simulink model "CDC_Library"  (R2015b)
settings: Solver=VariableStepAuto  StartTime=0  StopTime=1296000  RelTol=1e-3
InitFcn:
  | CD2_init
undefined symbols (not defined in the file): CD2_get_substances_count, table, tablestep
libraries: simulink x1
settings Model: Creator=garbanlo  LastModifiedBy=garbanlo
settings DataIOCC: LimitDataPoints=off  TimeSaveName=cd_time

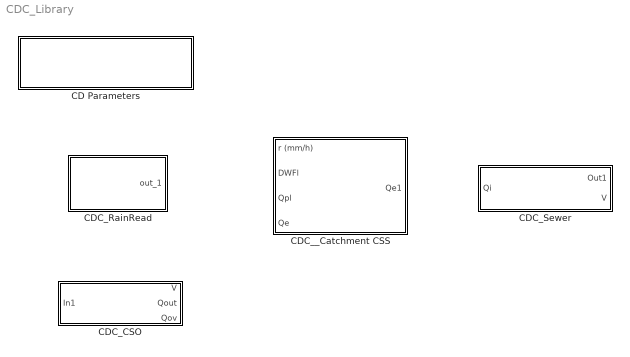
== system CDC_Library ==
  CD Parameters : Subsystem  mask(City Drain 2.0 - Simulation parameters){subst='COD HCO3 NH4', t_step=0, t_start=0, t_stop=15*24*60*60}
      mask prompts: subst "Modell Substances list (string)"; t_step "Sampling Time [s]"; t_start "Start Time [s]"; t_stop "Stop Time [s]"
      mask help:
      | Block that sets the global parameters required in City Drain 2.0. Following paramters are set without user's input:
      |
      | - 'Solver' --> 'FixedStepDiscrete'
      | - 'TimeSaveName' --> 'cd_time'
      | - 'Decimation' --> '1'
      | - 'LimitDataPoints' -->  'off'
      mask init:
      | % toplevel systems' name --> Plant file name;
      | tls=bdroot(gcb); 
      | %set_param(tls, 'Solver', 'FixedStepDiscrete'); 
      | set_param(tls, 'TimeSaveName', 'cd_time');
      | set_param(tls, 'Decimation', '1');
      | set_param(tls, 'LimitDataPoints', 'off');
      | set_param(tls, 'ScreenColor', 'white');
      | 
      | %tstep_char=num2str(t_step); % Setting the discrete time step
      | % set_param(tls, 'FixedStep', tstep_char); 
      | 
      | tstart_char=num2str(t_start); % Setting the start time
      | set_param(tls, 'StartTime', tstart_char); 
      | 
      | tstop_char=num2str(t_stop); % Setting the stop time
      | set_param(tls, 'StopTime', tstop_char);
      | 
      | set_param(gcs,'InitFcn','CD2_init');
      mask Display:
      | plot(0,0,100,100);
      | 
      | text(50,65,'CITY DRAIN','HorizontalAlignment','center');
      | text(50,35,'PARAMETERS','HorizontalAlignment','center');
      | 
      | 
      | image(imread('CityDrain_SimParam.jpg'))
  CDC_CSO : Subsystem  mask{Qout=0.02, V=1000, n_comp=CD2_get_substances_count}
      mask prompts: Qout "maximum outflow"; V "volume [m^3]"; n_comp "number of pollutants"
  CDC_RainRead : Subsystem  mask(Rain Read){table0='rainPulse5min.ixx', crep=off}
      mask prompts: table0 "Filename"; crep "Cylic repitition"
      mask help:
      | Read raindata from ASCII File in following formats:
      |
      | *.ixx ... Format used by the Austrian Hydrographic Service.
      | *.km2 ... Format used in the Mouse Software from DHI (Danish Hydraulic Institute)
      | *.mse ... modified mse format used in  Mouse Software from DHI (Danish Hydraulic Institute)
      |
      | Used function: CD1_mfun_rainread.m
      mask init:
      | % cache table size set to 1000
      | %table=zeros(1000,2)
      | [table,tablestep]=CD1_mfun_rainread(table0);
      | 
      | % reading the toplevel systems' name 
      | % --> Plant file name;
      | tls=bdroot(gcb); 
      | % Obtaining the fixed sampling time
      | % t_samp_char=get_param(tls, 'FixedStep');
      | % Convertion to numeric value
      | tstep = -1;
      mask Display:
      | plot(0,0,100,100);
      | 
      | text(40,40,'RAIN READ');
      | plot( [5 10 10 15 15 20 20 25 25 30 30 40 40 45], [0 0 20 20 40 40 60 60 30 30 0 0 0 0]+20);
  CDC_Sewer : Subsystem  mask(Sewer){K=300, alpha=0.5, n_comp=CD2_get_substances_count, beta=0.0001}
      mask prompts: K "K (travel time) [s]"; alpha "alpha (weighing factor,  0-1)  [ - ]"; n_comp "Number of pollutants [ - ]"; beta "beta (weighting factor)"
      mask help:
      | Function used:
      | CD1_sfun_Muskingum_Sewer.m
      mask init:
      | %arrow location in icon
      | kx=70;
      | ky=25;
      | % picture location
      | x=20;y=25;
      | 
      | 
      | % reading the toplevel systems' name 
      | % --> Plant file name;
      | % tls=bdroot(gcb); 
      | % Obtaining the fixed sampling time
      | % t_samp_char=get_param(tls, 'FixedStep');
      | % Convertion to numeric value
      | % dt = str2num(t_samp_char); 
      | tstep = -11
      mask Display:
      | plot(0,0,100,50, [0,50,50,0,0]+x,[-10,-10,10,10,-10]+y, [10,10]+x,[-10,10]+y, [20,20]+x,[-10,10]+y, [30,30]+x,[-10,10]+y, [40,40]+x,[-10,10]+y, [0,0,5,5,10,5,5,0]+kx, [5,-5,-5,-13,0,13,5,5]+ky );
      | 
      | 
      | text(50,7,'SEWER sM','HorizontalAlignment','center');
      | 
      | port_label('input',1,'Qi');
      | port_label('output',1,'Qe');
      | port_label('output',2,'VCi');
  CDC__Catchment CSS : Subsystem  mask(Catchment CSS){area=2, rfcoeff=0.5, initloss=1.5, permloss=1.25, N=3, n_comp=CD2_get_substances_count, Rain_C=[2 0 0], K=300, X=0}
      mask prompts: area "Area in [ha]"; rfcoeff "Runoff coefficient (0 - 1)"; initloss "Initial Loss in [mm]"; permloss "Permanent loss in [mm/day]"; N "No of Timesteps (transport time) / No of subareas n [-]"; n_comp "No of pollutant components"; Rain_C "Vector of Rain-Conc. [g/m3]"
      mask help:
      | Hydrological model of an urban catchment with a combined sewer system.
      | --> see manual for more details
      mask init:
      | % location of catchment drawing
      | x=10;
      | y=-10;
      | % reading the toplevel systems' name 
      | % --> Plant file name;
      | tls=bdroot(gcb); 
      | % Obtaining the fixed sampling time
      | % t_samp_char=get_param(tls, 'FixedStep');
      | 
      | % Convertion to numeric value
      | % tstep = str2num(t_samp_char); 
      | tstep = 60;
      | 
      | %convertion form mm/day --> mm/s
      | permloss=permloss/86400;
      | area=area*10000;
      | 
      | %parameter for muskingum
      | CX=(-K*X)/(K*(1-X));
      | CY=1/(K*(1-X));
      mask Display:
      | plot(0,0,100,100, [17 20 25 30 40 45 50 55 60 65]+x, [60 80 82 85 88 88 88 85 75 60]+y);
      | plot(0,0,100,100, [17 20 25 30 40 45 50 55 60 65]+x, [55 40 35 30 30 30 30 35 40 55]+y);
      | 
      | plot([20 65]+x,[60 60]+y);
      | plot([20 30]+x,[80 60]+y);
      | plot([30 40]+x,[75 60]+y);
      | plot([45 60]+x,[75 60]+y);
      | plot([20 65]+x,[55 55]+y);
      | plot([20 30]+x,[40 55]+y);
      | plot([30 40]+x,[45 55]+y);
      | plot([45 60]+x,[30 55]+y);
      | 
      | color('black');
      | 
      | port_label('input',1,'rl (mm/h)');
      | port_label('input',2,'DWFl (mg/l)');
      | port_label('input',3,'Qpl (mg/l)');
      | port_label('input',4,'Qe (mg/l!)');
      | port_label('output',1,'Qe(mg/s)');
      | 
      | text(50,90,'CATCHMENT CSS','HorizontalAlignment','center');

== system CDC_Library/CD Parameters ==

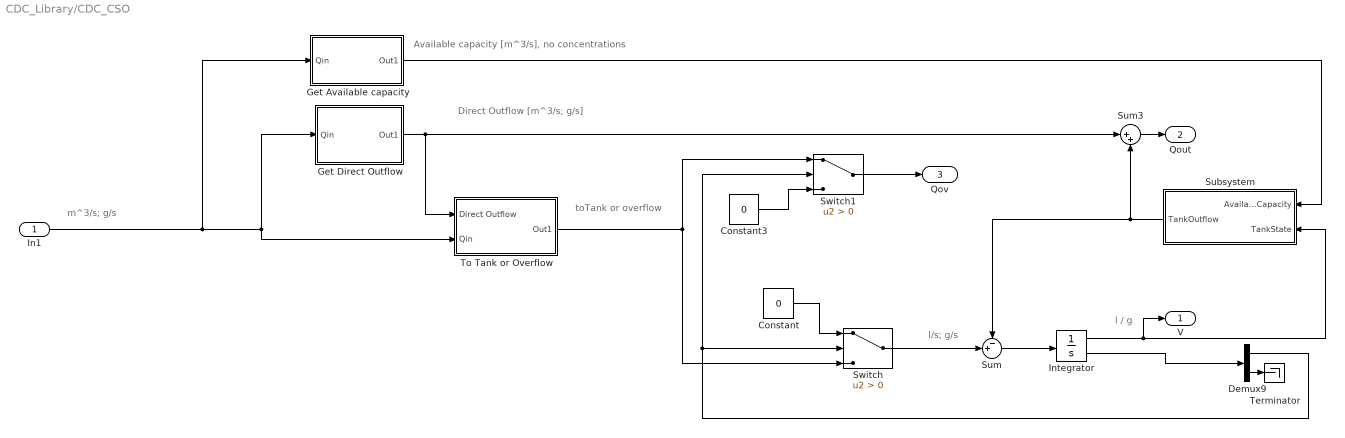
== system CDC_Library/CDC_CSO ==
  note: m^3/s; g/s
  note: Available capacity [m^3/s], no concentrations
  note: toTank or overflow
  note: Direct Outflow [m^3/s; g/s]
  note: l/s; g/s
  note: l / g
  In1 : Inport
  Constant : Constant  Value=0
  Constant3 : Constant  Value=0
  Demux9 : Demux  Outputs=[1,n_comp]
  Get Available capacity : Subsystem
  Get Direct Outflow : Subsystem
  Integrator : Integrator  InitialCondition=0.000001  LimitOutput=on  UpperSaturationLimit=1000  LowerSaturationLimit=0  ShowSaturationPort=on
  Subsystem : Subsystem
  Sum : Sum  Inputs=-+|
  Sum3 : Sum  Inputs=|++
  Switch : Switch  Criteria=u2 > Threshold
  Switch1 : Switch  Criteria=u2 > Threshold
  Terminator : Terminator
  To Tank or Overflow : Subsystem
  V : Outport
  Qout : Outport  Port=2
  Qov : Outport  Port=3
  wires:
  Sum/1 -> Integrator/1
  In1/1 -> Get Available capacity/1(Qin), Get Direct Outflow/1(Qin), To Tank or Overflow/2(Qin)
  Constant3/1 -> Switch1/3
  Sum3/1 -> Qout/1
  Get Available capacity/1(Out1) -> Subsystem/1(AvailableCapacity)
  Switch1/1 -> Qov/1
  Integrator/1 -> V/1, Subsystem/2(TankState)
  Get Direct Outflow/1(Out1) -> To Tank or Overflow/1(Direct Outflow), Sum3/1
  Subsystem/1(TankOutflow) -> Sum3/2, Sum/1
  Constant/1 -> Switch/1
  Switch/1 -> Sum/2
  Integrator/2 -> Demux9/1
  Demux9/1 -> Switch1/2, Switch/2
  Demux9/2 -> Terminator/1
  To Tank or Overflow/1(Out1) -> Switch/3, Switch1/1

== system CDC_Library/CDC_RainRead ==
  rainread : S-Function  FunctionName=CDC_sfun_rainread  Parameters=crep,table,tablestep,tstep  SFunctionDeploymentMode=off  EnableBusSupport=off
  out_1 : Outport
  wires:
  rainread/1 -> out_1/1

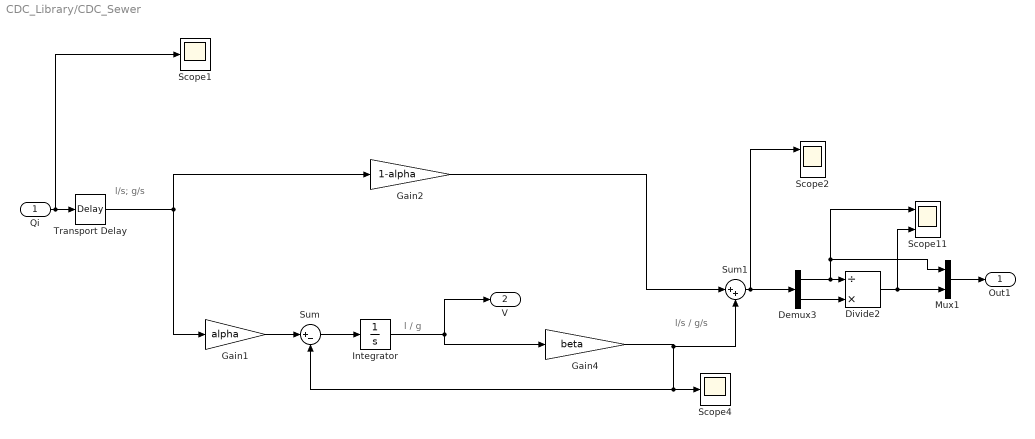
== system CDC_Library/CDC_Sewer ==
  note: l/s / g/s
  note: l / g
  note: l/s; g/s
  Qi : Inport
  Demux3 : Demux  Outputs=[1, n_comp]
  Divide2 : Product  Inputs=/*
  Gain1 : Gain  Gain=alpha
  Gain2 : Gain  Gain=1-alpha
  Gain4 : Gain  Gain=beta
  Integrator : Integrator  InitialCondition=0.000001  LimitOutput=on  LowerSaturationLimit=0
  Mux1 : Mux  Inputs=2
  Scope1 : Scope
  Scope11 : Scope  NumInputPorts=2
  Scope2 : Scope  NumInputPorts=2
  Scope4 : Scope
  Sum : Sum  Inputs=|+-
  Sum1 : Sum  Inputs=|++
  Transport Delay : TransportDelay
  Out1 : Outport
  V : Outport  Port=2
  wires:
  Qi/1 -> Scope1/1, Transport Delay/1
  Integrator/1 -> Gain4/1, V/1
  Sum/1 -> Integrator/1
  Transport Delay/1 -> Gain2/1, Gain1/1
  Gain1/1 -> Sum/1
  Gain2/1 -> Sum1/1
  Mux1/1 -> Out1/1
  Demux3/1 -> Mux1/1, Scope11/1, Divide2/1
  Demux3/2 -> Divide2/2
  Divide2/1 -> Mux1/2, Scope11/2
  Gain4/1 -> Sum1/2, Sum/2, Scope4/1
  Sum1/1 -> Scope2/1, Demux3/1

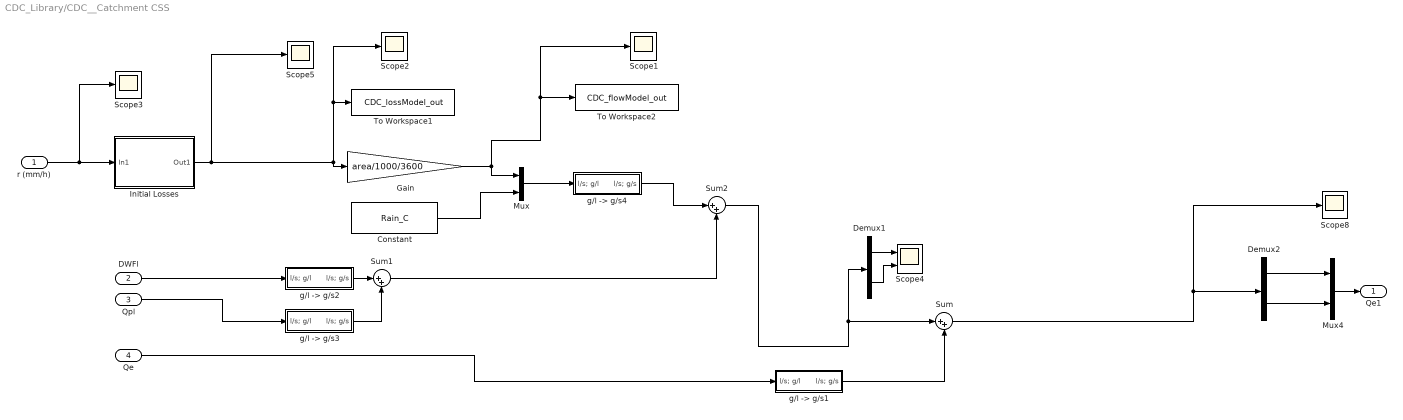
== system CDC_Library/CDC__Catchment CSS ==
  r (mm/h) : Inport
  DWFl : Inport  Port=2
  Qpl : Inport  Port=3
  Qe : Inport  Port=4
  Constant : Constant  Value=Rain_C
  Demux1 : Demux  Outputs=[1, n_comp]
  Demux2 : Demux  Outputs=[1, n_comp]
  Gain : Gain  Gain=area/1000/3600
  Initial Losses : Subsystem
  Mux : Mux  Inputs=2
  Mux4 : Mux  Inputs=[1, n_comp]
  Scope{1..3,5,8} (5 alike) : Scope
  Scope4 : Scope  NumInputPorts=2
  Sum : Sum  Inputs=|++
  Sum1 : Sum  Inputs=|++
  Sum2 : Sum  Inputs=|++
  To Workspace1 : ToWorkspace  VariableName=CDC_lossModel_out  SaveFormat=Timeseries  SampleTime=-1
  To Workspace2 : ToWorkspace  VariableName=CDC_flowModel_out  SaveFormat=Timeseries  SampleTime=-1
  "g/l -> g/s1" : Subsystem
  "g/l -> g/s2" : Subsystem
  "g/l -> g/s3" : Subsystem
  "g/l -> g/s4" : Subsystem
  Qe1 : Outport
  wires:
  Mux/1 -> "g/l -> g/s4"/1(l/s; g/l)
  DWFl/1 -> "g/l -> g/s2"/1(l/s; g/l)
  Qpl/1 -> "g/l -> g/s3"/1(l/s; g/l)
  r (mm/h)/1 -> Scope3/1, Initial Losses/1(In1)
  Gain/1 -> Scope1/1, To Workspace2/1, Mux/1
  Constant/1 -> Mux/2
  Demux2/1 -> Mux4/1
  Mux4/1 -> Qe1/1
  Demux2/2 -> Mux4/2
  Initial Losses/1(Out1) -> Scope5/1, Gain/1, Scope2/1, To Workspace1/1
  Sum/1 -> Demux2/1, Scope8/1
  Qe/1 -> "g/l -> g/s1"/1(l/s; g/l)
  "g/l -> g/s1"/1(l/s; g/s) -> Sum/2
  Sum2/1 -> Demux1/1, Sum/1
  Demux1/1 -> Scope4/1
  Demux1/2 -> Scope4/2
  "g/l -> g/s2"/1(l/s; g/s) -> Sum1/1
  "g/l -> g/s3"/1(l/s; g/s) -> Sum1/2
  "g/l -> g/s4"/1(l/s; g/s) -> Sum2/1
  Sum1/1 -> Sum2/2

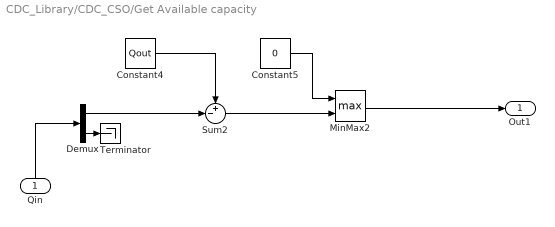
== system CDC_Library/CDC_CSO/Get Available capacity ==
  Qin : Inport
  Constant4 : Constant  Value=Qout
  Constant5 : Constant  Value=0
  Demux : Demux  Outputs=[1,n_comp]
  MinMax2 : MinMax  Function=max  Inputs=2
  Sum2 : Sum  Inputs=+-|
  Terminator : Terminator
  Out1 : Outport
  wires:
  Constant5/1 -> MinMax2/1
  Constant4/1 -> Sum2/1
  MinMax2/1 -> Out1/1
  Sum2/1 -> MinMax2/2
  Demux/1 -> Sum2/2
  Qin/1 -> Demux/1
  Demux/2 -> Terminator/1

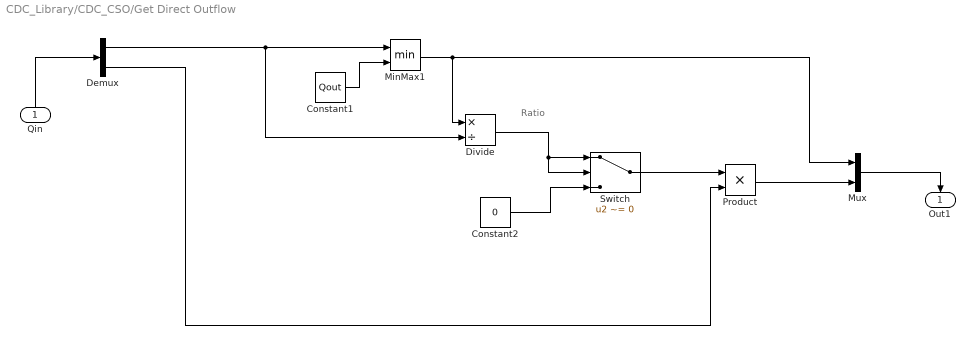
== system CDC_Library/CDC_CSO/Get Direct Outflow ==
  note: Ratio
  Qin : Inport
  Constant1 : Constant  Value=Qout
  Constant2 : Constant  Value=0
  Demux : Demux  Outputs=[1,n_comp]
  Divide : Product  Inputs=*/
  MinMax1 : MinMax  Inputs=2
  Mux : Mux  Inputs=2
  Product : Product
  Switch : Switch  Criteria=u2 ~= 0
  Out1 : Outport
  wires:
  MinMax1/1 -> Mux/1, Divide/1
  Constant1/1 -> MinMax1/2
  Qin/1 -> Demux/1
  Demux/1 -> Divide/2, MinMax1/1
  Demux/2 -> Product/2
  Product/1 -> Mux/2
  Mux/1 -> Out1/1
  Divide/1 -> Switch/2, Switch/1
  Switch/1 -> Product/1
  Constant2/1 -> Switch/3

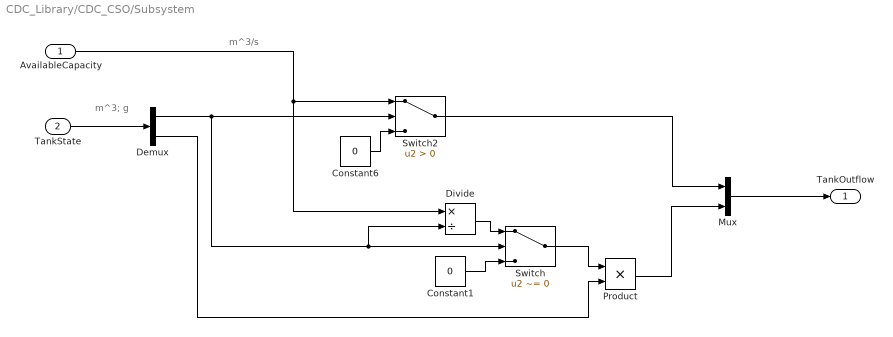
== system CDC_Library/CDC_CSO/Subsystem ==
  note: m^3; g
  note: m^3/s
  AvailableCapacity : Inport
  TankState : Inport  Port=2
  Constant1 : Constant  Value=0
  Constant6 : Constant  Value=0
  Demux : Demux  Outputs=[1,n_comp]
  Divide : Product  Inputs=*/
  Mux : Mux  Inputs=2
  Product : Product
  Switch : Switch  Criteria=u2 ~= 0
  Switch2 : Switch  Criteria=u2 > Threshold
  TankOutflow : Outport
  wires:
  AvailableCapacity/1 -> Switch2/1, Divide/1
  Constant6/1 -> Switch2/3
  TankState/1 -> Demux/1
  Demux/2 -> Product/2
  Demux/1 -> Switch2/2, Switch/2, Divide/2
  Divide/1 -> Switch/1
  Constant1/1 -> Switch/3
  Switch/1 -> Product/1
  Product/1 -> Mux/2
  Switch2/1 -> Mux/1
  Mux/1 -> TankOutflow/1

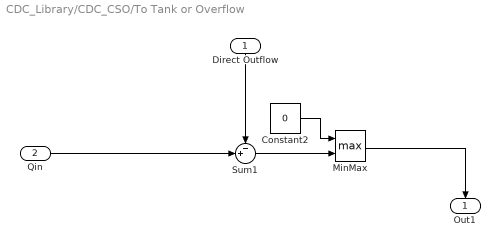
== system CDC_Library/CDC_CSO/To Tank or Overflow ==
  Direct Outflow : Inport
  Qin : Inport  Port=2
  Constant2 : Constant  Value=0
  MinMax : MinMax  Function=max  Inputs=2
  Sum1 : Sum  Inputs=-+|
  Out1 : Outport
  wires:
  Constant2/1 -> MinMax/1
  Sum1/1 -> MinMax/2
  MinMax/1 -> Out1/1
  Direct Outflow/1 -> Sum1/1
  Qin/1 -> Sum1/2

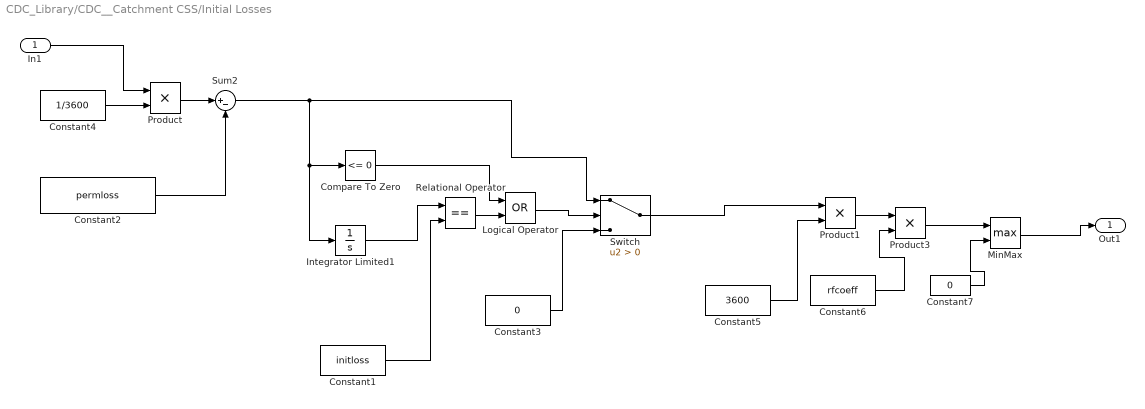
== system CDC_Library/CDC__Catchment CSS/Initial Losses ==
  In1 : Inport
  Compare To Zero : simulink/Logic and Bit Operations/Compare To Zero  relop=<=  OutDataTypeStr=boolean
  Constant1 : Constant  Value=initloss
  Constant2 : Constant  Value=permloss
  Constant3 : Constant  Value=0
  Constant4 : Constant  Value=1/3600
  Constant5 : Constant  Value=3600
  Constant6 : Constant  Value=rfcoeff
  Constant7 : Constant  Value=0
  Integrator Limited1 : Integrator  LimitOutput=on  UpperSaturationLimit=initloss  LowerSaturationLimit=0
  Logical Operator : Logic  Operator=OR  AllPortsSameDT=off  OutDataTypeStr=boolean
  MinMax : MinMax  Function=max  Inputs=2
  Product : Product
  Product1 : Product
  Product3 : Product
  Relational Operator : RelationalOperator  Operator===  OutDataTypeStr=boolean
  Sum2 : Sum  Inputs=|+-
  Switch : Switch  Criteria=u2 > Threshold
  Out1 : Outport
  wires:
  Integrator Limited1/1 -> Relational Operator/1
  Constant1/1 -> Relational Operator/2
  Constant2/1 -> Sum2/2
  Sum2/1 -> Integrator Limited1/1, Compare To Zero/1, Switch/1
  Constant3/1 -> Switch/3
  Product/1 -> Sum2/1
  Constant4/1 -> Product/2
  Relational Operator/1 -> Logical Operator/2
  Logical Operator/1 -> Switch/2
  Compare To Zero/1 -> Logical Operator/1
  Constant5/1 -> Product1/2
  Switch/1 -> Product1/1
  Product1/1 -> Product3/1
  Product3/1 -> MinMax/1
  Constant6/1 -> Product3/2
  MinMax/1 -> Out1/1
  Constant7/1 -> MinMax/2
  In1/1 -> Product/1

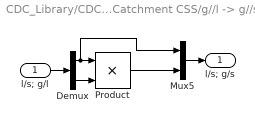
== system CDC_Library/CDC__Catchment CSS/g//l -> g//s1 ==
  l/s; g/l : Inport
  Demux : Demux  Outputs=[1, n_comp]
  Mux5 : Mux  Inputs=2
  Product : Product
  l/s; g/s : Outport
  wires:
  Product/1 -> Mux5/2
  Demux/2 -> Product/2
  Demux/1 -> Mux5/1, Product/1
  Mux5/1 -> l/s; g/s/1
  l/s; g/l/1 -> Demux/1

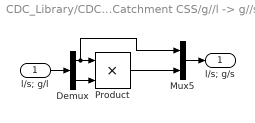
== system CDC_Library/CDC__Catchment CSS/g//l -> g//s2 ==
  l/s; g/l : Inport
  Demux : Demux  Outputs=[1, n_comp]
  Mux5 : Mux  Inputs=2
  Product : Product
  l/s; g/s : Outport
  wires:
  Product/1 -> Mux5/2
  Demux/2 -> Product/2
  Demux/1 -> Mux5/1, Product/1
  Mux5/1 -> l/s; g/s/1
  l/s; g/l/1 -> Demux/1

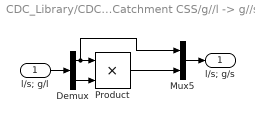
== system CDC_Library/CDC__Catchment CSS/g//l -> g//s3 ==
  l/s; g/l : Inport
  Demux : Demux  Outputs=[1, n_comp]
  Mux5 : Mux  Inputs=2
  Product : Product
  l/s; g/s : Outport
  wires:
  Product/1 -> Mux5/2
  Demux/2 -> Product/2
  Demux/1 -> Mux5/1, Product/1
  Mux5/1 -> l/s; g/s/1
  l/s; g/l/1 -> Demux/1

== system CDC_Library/CDC__Catchment CSS/g//l -> g//s4 ==
  l/s; g/l : Inport
  Demux : Demux  Outputs=[1, n_comp]
  Mux5 : Mux  Inputs=2
  Product : Product
  l/s; g/s : Outport
  wires:
  Product/1 -> Mux5/2
  Demux/2 -> Product/2
  Demux/1 -> Mux5/1, Product/1
  Mux5/1 -> l/s; g/s/1
  l/s; g/l/1 -> Demux/1
